simulink model "foc_7"  (R2024a)
settings: Solver=FixedStepAuto  StartTime=0.0  StopTime=3  FixedStep=1e-6  MaxStep=1e-5  RelTol=1e-3
undefined symbols (not defined in the file): DiscIntNeverNeededParam, Ki, Ki_s, Kp, Kp_s, L, lambda, ma, p, R, T_period, Vdc
libraries: simulink x13, spsIGBTDiodeLib x6, spsSeriesRLCBranchLib x6, eeGeneralControl x6, spsCurrentMeasurementLib x3, spsPermanentMagnetSynchronousMachineLib x2, spsDCVoltageSourceLib x1, spsStairGeneratorLib x1, spspowerguiLib x1
(part 2 of 2)

== system foc_7/Subsystem2/Subsystem5/Limitations ==
  Vq_ref1 : Inport
  Vd_ref1 : Inport  Port=2
  Action Port : ActionPort  ActionPortLabel=else
  Add : Sum
  Gain : Gain  Gain=sqrt(3)
  Gain1 : Gain  Gain=Vdc*ma
  Gain2 : Gain  Gain=Vdc*ma
  Product : Product  Inputs=*/
  Product1 : Product  Inputs=/*
  Sqrt : Sqrt
  Square : Math  Operator=square  SignedPower=on
  Square1 : Math  Operator=square  SignedPower=on
  Vq_ref2 : Outport
  Vd_ref2 : Outport  Port=2
  wires:
  Vq_ref1/1 -> Gain2/1, Square/1
  Vd_ref1/1 -> Gain1/1, Square1/1
  Square/1 -> Add/1
  Square1/1 -> Add/2
  Add/1 -> Sqrt/1
  Sqrt/1 -> Gain/1
  Gain2/1 -> Product/1
  Gain1/1 -> Product1/2
  Gain/1 -> Product/2, Product1/1
  Product/1 -> Vq_ref2/1
  Product1/1 -> Vd_ref2/1

== system foc_7/Subsystem2/Subsystem5/Linear Operation  ==
  Vq_ref1 : Inport
  Vd_ref1 : Inport  Port=2
  Action Port : ActionPort  ActionPortLabel=if(u1 <= 0)
  Vq_ref2 : Outport
  Vd_ref2 : Outport  Port=2
  wires:
  Vq_ref1/1 -> Vq_ref2/1
  Vd_ref1/1 -> Vd_ref2/1

== system foc_7/Subsystem3/SVPWM/ABC to alpha-beta ==
  In1 : Inport
  In2 : Inport  Port=2
  In3 : Inport  Port=3
  Add : Sum  Inputs=+--
  Add1 : Sum  Inputs=+-
  Gain : Gain  Gain=0.5
  Gain1 : Gain  Gain=0.5
  Gain2 : Gain  Gain=2/3
  Gain3 : Gain  Gain=sqrt(3)/2
  Gain4 : Gain  Gain=sqrt(3)/2
  Gain5 : Gain  Gain=2/3
  Scope1 : Scope  NumInputPorts=3
  alpha : Outport
  beta : Outport  Port=2
  wires:
  Gain3/1 -> Add1/1
  In2/1 -> Gain3/1, Scope1/2, Gain/1
  Gain4/1 -> Add1/2
  Add1/1 -> Gain5/1
  Gain1/1 -> Add/3
  In3/1 -> Scope1/3, Gain4/1, Gain1/1
  Gain/1 -> Add/2
  In1/1 -> Add/1, Scope1/1
  Add/1 -> Gain2/1
  Gain2/1 -> alpha/1  "alpha"
  Gain5/1 -> beta/1  "beta"

== system foc_7/Subsystem3/SVPWM/PWM ==
  ref1 : Inport
  ref2 : Inport  Port=2
  ref3 : Inport  Port=3
  Carrier : Inport  Port=4
  Relational Operator : RelationalOperator  OutDataTypeStr=boolean  RndMeth=Simplest  InputSameDT=off
  Relational Operator1 : RelationalOperator  OutDataTypeStr=boolean  RndMeth=Simplest  InputSameDT=off
  Relational Operator2 : RelationalOperator  OutDataTypeStr=boolean  RndMeth=Simplest  InputSameDT=off
  PWM1 : Outport
  PWM3 : Outport  Port=2
  PWM5 : Outport  Port=3
  wires:
  ref1/1 -> Relational Operator/1
  ref2/1 -> Relational Operator1/1
  ref3/1 -> Relational Operator2/1
  Carrier/1 -> Relational Operator/2, Relational Operator2/2, Relational Operator1/2
  Relational Operator/1 -> PWM1/1
  Relational Operator1/1 -> PWM3/1
  Relational Operator2/1 -> PWM5/1

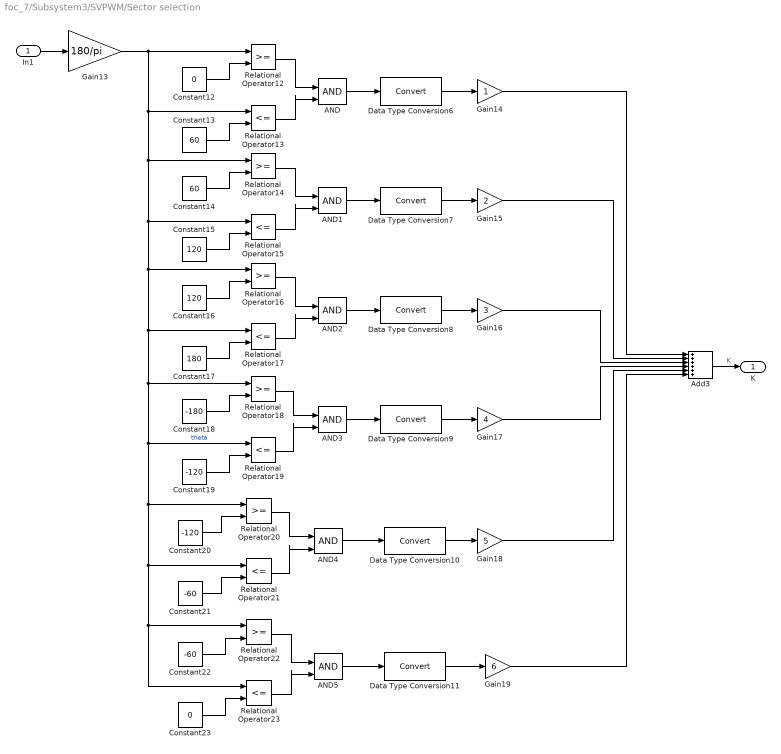
== system foc_7/Subsystem3/SVPWM/Sector selection ==
  In1 : Inport
  AND{,1..5} (6 alike) : Logic  IconShape=distinctive  AllPortsSameDT=off  OutDataTypeStr=boolean
  Add3 : Sum  Inputs=++++++
  Constant12 : Constant  Value=0
  Constant13 : Constant  Value=60
  Constant14 : Constant  Value=60
  Constant15 : Constant  Value=120
  Constant16 : Constant  Value=120
  Constant17 : Constant  Value=180
  Constant18 : Constant  Value=-180
  Constant19 : Constant  Value=-120
  Constant20 : Constant  Value=-120
  Constant21 : Constant  Value=-60
  Constant22 : Constant  Value=-60
  Constant23 : Constant  Value=0
  Data Type Conversion{6..11} (6 alike) : DataTypeConversion  SaturateOnIntegerOverflow=off  RndMeth=Floor
  Gain13 : Gain  Gain=180/pi
  Gain14 : Gain
  Gain15 : Gain  Gain=2
  Gain16 : Gain  Gain=3
  Gain17 : Gain  Gain=4
  Gain18 : Gain  Gain=5
  Gain19 : Gain  Gain=6
  Relational Operator{12,14,16,18,20,22} (6 alike) : RelationalOperator  OutDataTypeStr=boolean  RndMeth=Simplest  InputSameDT=off
  Relational Operator{13,15,17,19,21,23} (6 alike) : RelationalOperator  Operator=<=  OutDataTypeStr=boolean  RndMeth=Simplest  InputSameDT=off
  K : Outport
  wires:
  AND2/1 -> Data Type Conversion8/1
  Relational Operator14/1 -> AND1/1
  Relational Operator12/1 -> AND/1
  Data Type Conversion10/1 -> Gain18/1
  Data Type Conversion8/1 -> Gain16/1
  Relational Operator19/1 -> AND3/2
  Gain13/1 -> Relational Operator14/1, Relational Operator18/1, Relational Operator19/1, Relational Operator20/1, Relational Operator22/1, Relational Operator23/1, Relational Operator21/1, Relational Operator17/1, Relational Operator16/1, Relational Operator15/1, Relational Operator13/1, Relational Operator12/1  "theta"
  Data Type Conversion6/1 -> Gain14/1
  Constant21/1 -> Relational Operator21/2
  Constant19/1 -> Relational Operator19/2
  Gain19/1 -> Add3/6
  Constant18/1 -> Relational Operator18/2
  AND4/1 -> Data Type Conversion10/1
  Constant22/1 -> Relational Operator22/2
  Relational Operator22/1 -> AND5/1
  Relational Operator18/1 -> AND3/1
  Gain15/1 -> Add3/2
  Relational Operator23/1 -> AND5/2
  Data Type Conversion11/1 -> Gain19/1
  Constant16/1 -> Relational Operator16/2
  Data Type Conversion7/1 -> Gain15/1
  Constant23/1 -> Relational Operator23/2
  Relational Operator20/1 -> AND4/1
  Gain18/1 -> Add3/5
  Gain14/1 -> Add3/1
  AND1/1 -> Data Type Conversion7/1
  Constant14/1 -> Relational Operator14/2
  Relational Operator16/1 -> AND2/1
  Relational Operator17/1 -> AND2/2
  Gain17/1 -> Add3/4
  Constant12/1 -> Relational Operator12/2
  Gain16/1 -> Add3/3
  Relational Operator13/1 -> AND/2
  Relational Operator15/1 -> AND1/2
  Data Type Conversion9/1 -> Gain17/1
  AND/1 -> Data Type Conversion6/1
  Constant13/1 -> Relational Operator13/2
  Relational Operator21/1 -> AND4/2
  AND3/1 -> Data Type Conversion9/1
  Constant20/1 -> Relational Operator20/2
  Constant17/1 -> Relational Operator17/2
  AND5/1 -> Data Type Conversion11/1
  Constant15/1 -> Relational Operator15/2
  Add3/1 -> K/1  "K"
  In1/1 -> Gain13/1

== system foc_7/Subsystem3/SVPWM/Subsystem3 ==
  In1 : Inport
  In2 : Inport  Port=2
  In3 : Inport  Port=3
  Add10 : Sum
  Add8 : Sum  Inputs=+++
  Add9 : Sum
  Gain{9..12} (4 alike) : Gain  Gain=0.5
  S1 : Outport
  S3 : Outport  Port=2
  S6 : Outport  Port=3
  S5 : Outport  Port=4
  wires:
  In3/1 -> Gain9/1, Gain10/1, Gain12/1, Gain11/1
  Gain11/1 -> Add10/2
  Gain9/1 -> Add8/3
  Gain10/1 -> Add9/2
  Add8/1 -> S1/1  "S1"
  In2/1 -> Add9/1, Add8/2
  In1/1 -> Add10/1, Add8/1
  Add9/1 -> S3/1  "S3"
  Gain12/1 -> S5/1  "S5"
  Add10/1 -> S6/1  "S6"

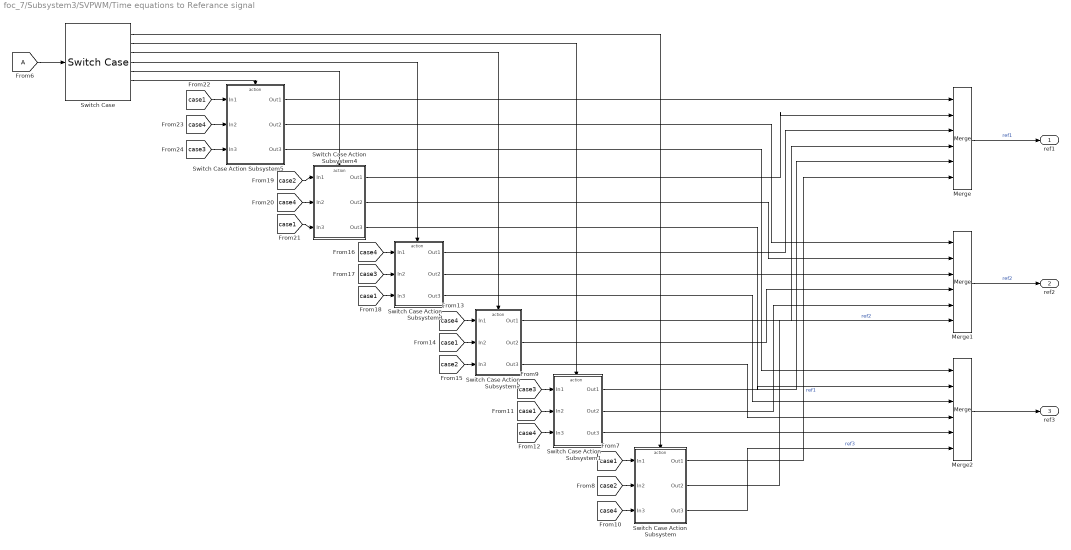
== system foc_7/Subsystem3/SVPWM/Time equations to Referance signal ==
  From6 : From  TagVisibility=global
  Merge : Merge  Inputs=6
  Merge1 : Merge  Inputs=6
  Merge2 : Merge  Inputs=6
  Switch Case : SwitchCase  CaseConditions={1 2 3 4 5 6}
  Switch Case Action Subsystem : Subsystem  TreatAsAtomicUnit=on
  Switch Case Action Subsystem1 : Subsystem  TreatAsAtomicUnit=on
  Switch Case Action Subsystem2 : Subsystem  TreatAsAtomicUnit=on
  Switch Case Action Subsystem3 : Subsystem  TreatAsAtomicUnit=on
  Switch Case Action Subsystem4 : Subsystem  TreatAsAtomicUnit=on
  Switch Case Action Subsystem5 : Subsystem  TreatAsAtomicUnit=on
  ref1 : Outport
  "ref2 " : Outport  Port=2
  ref3 : Outport  Port=3
  wires:
  [case3] -> Switch Case Action Subsystem5/3(In3)
  Switch Case Action Subsystem4/1(Out1) -> Merge/2
  [case1] -> Switch Case Action Subsystem2/2(In2)
  Switch Case Action Subsystem3/2(Out2) -> Merge1/3
  [case4] -> Switch Case Action Subsystem3/1(In1)
  Switch Case/4 -> Switch Case Action Subsystem3/Action
  [case2] -> Switch Case Action Subsystem4/1(In1)
  Switch Case/6 -> Switch Case Action Subsystem5/Action
  [case4] -> Switch Case Action Subsystem1/3(In3)
  [case1] -> Switch Case Action Subsystem5/1(In1)
  [case3] -> Switch Case Action Subsystem1/1(In1)
  Merge/1 -> ref1/1  "ref1"
  Switch Case Action Subsystem5/1(Out1) -> Merge/1
  Switch Case/5 -> Switch Case Action Subsystem4/Action
  Switch Case Action Subsystem4/3(Out3) -> Merge2/2
  [case1] -> Switch Case Action Subsystem/1(In1)
  Switch Case Action Subsystem2/3(Out3) -> Merge2/4
  Switch Case Action Subsystem4/2(Out2) -> Merge1/2
  Switch Case/3 -> Switch Case Action Subsystem2/Action
  Switch Case Action Subsystem/2(Out2) -> Merge1/6  "ref2"
  Switch Case Action Subsystem3/3(Out3) -> Merge2/3
  Switch Case Action Subsystem5/2(Out2) -> Merge1/1
  [case3] -> Switch Case Action Subsystem3/2(In2)
  Switch Case/2 -> Switch Case Action Subsystem1/Action
  Switch Case Action Subsystem2/1(Out1) -> Merge/4
  Switch Case Action Subsystem2/2(Out2) -> Merge1/4
  [case1] -> Switch Case Action Subsystem4/3(In3)
  [case4] -> Switch Case Action Subsystem5/2(In2)
  Switch Case/1 -> Switch Case Action Subsystem/Action
  Switch Case Action Subsystem5/3(Out3) -> Merge2/1
  [case4] -> Switch Case Action Subsystem2/1(In1)
  Switch Case Action Subsystem3/1(Out1) -> Merge/3
  [case4] -> Switch Case Action Subsystem/3(In3)
  Merge2/1 -> ref3/1
  From6/1 -> Switch Case/1
  [case4] -> Switch Case Action Subsystem4/2(In2)
  [case2] -> Switch Case Action Subsystem/2(In2)
  [case2] -> Switch Case Action Subsystem2/3(In3)
  [case1] -> Switch Case Action Subsystem3/3(In3)
  Switch Case Action Subsystem1/2(Out2) -> Merge1/5
  Switch Case Action Subsystem/1(Out1) -> Merge/6  "ref1"
  Switch Case Action Subsystem1/1(Out1) -> Merge/5
  Switch Case Action Subsystem/3(Out3) -> Merge2/6  "ref3"
  Switch Case Action Subsystem1/3(Out3) -> Merge2/5
  [case1] -> Switch Case Action Subsystem1/2(In2)
  Merge1/1 -> "ref2 "/1  "ref2"

== system foc_7/Subsystem3/SVPWM/polar form ==
  In1 : Inport
  In2 : Inport  Port=2
  Add2 : Sum
  Atan2 : Trigonometry  Operator=atan2
  Math Function : Math  Operator=square  SignedPower=on
  Math Function1 : Math  Operator=square  SignedPower=on
  Saturation2 : Saturate  UpperLimit=0.95 * Vdc /sqrt(3)  LowerLimit=0
  Scope1 : Scope  NumInputPorts=2
  Scope2 : Scope  NumInputPorts=2
  Square Root : Sqrt
  Vr : Outport
  Angle : Outport  Port=2
  wires:
  In2/1 -> Scope2/2, Atan2/2, Math Function1/1
  In1/1 -> Scope2/1, Atan2/1, Math Function/1
  Math Function1/1 -> Add2/2
  Add2/1 -> Square Root/1
  Math Function/1 -> Add2/1
  Atan2/1 -> Angle/1
  Square Root/1 -> Saturation2/1, Scope1/1  "Vr"
  Saturation2/1 -> Vr/1, Scope1/2

== system foc_7/Subsystem3/SVPWM/time equations ==
  Vref : Inport
  Sector : Inport  Port=2
  Angle : Inport  Port=3
  Add4 : Sum  Inputs=+-
  Add5 : Sum  Inputs=+-
  Add6 : Sum  Inputs=+-
  Add7 : Sum  Inputs=+--
  Constant : Constant  Value=T_period
  Divide : Product  Inputs=*/
  Gain6 : Gain  Gain=sqrt(3)*(T_period)
  Gain7 : Gain  Gain=pi/3
  Gain8 : Gain  Gain=pi/3
  Product : Product
  Product1 : Product
  Sin1 : Trigonometry
  Sin4 : Trigonometry
  Vdc : Constant  Value=Vdc
  const : Constant
  T1 : Outport
  T2 : Outport  Port=2
  T0 : Outport  Port=3
  wires:
  Vdc/1 -> Divide/2
  Gain6/1 -> Product1/1, Product/1
  Divide/1 -> Gain6/1
  Add6/1 -> Gain8/1
  Constant/1 -> Add7/1
  Gain7/1 -> Add4/1
  Add5/1 -> Sin4/1
  Sin4/1 -> Product1/2
  Sin1/1 -> Product/2
  Gain8/1 -> Add5/2
  Angle/1 -> Add5/1, Add4/2
  const/1 -> Add6/2
  Product1/1 -> T2/1, Add7/3  "T2"
  Sector/1 -> Gain7/1, Add6/1
  Add4/1 -> Sin1/1
  Vref/1 -> Divide/1
  Product/1 -> Add7/2, T1/1  "T1"
  Add7/1 -> T0/1

== system foc_7/Subsystem3/Subsystem2/PI_Controller_Id ==
  Id_error : Inport
  Discrete-Time Integrator1 : DiscreteIntegrator  SampleTime=-1  ICPrevOutput=DiscIntNeverNeededParam  ICPrevScaledInput=DiscIntNeverNeededParam
  Gain1 : Gain  Gain=Kp
  Gain2 : Gain  Gain=Ki
  Product : Product
  Scope : Scope  NumInputPorts=2
  Scope1 : Scope
  Sum1 : Sum
  Vd_coupled : Outport
  wires:
  [Stop_d_integrator] -> Scope/2, Product/1
  Sum1/1 -> Scope1/1, Vd_coupled/1
  Product/1 -> Scope/1, Discrete-Time Integrator1/1
  Gain2/1 -> Product/2
  Discrete-Time Integrator1/1 -> Sum1/2
  Gain1/1 -> Sum1/1
  Id_error/1 -> Gain2/1, Gain1/1

== system foc_7/Subsystem3/Subsystem2/PI_Controller_Iq ==
  Iq_error : Inport
  Discrete-Time Integrator1 : DiscreteIntegrator  SampleTime=-1  ICPrevOutput=DiscIntNeverNeededParam  ICPrevScaledInput=DiscIntNeverNeededParam
  Gain1 : Gain  Gain=Kp
  Gain2 : Gain  Gain=Ki
  Product : Product
  Scope : Scope  NumInputPorts=2
  Scope1 : Scope
  Sum1 : Sum
  Vq_coupled : Outport
  wires:
  Product/1 -> Scope/1, Discrete-Time Integrator1/1
  Iq_error/1 -> Gain2/1, Gain1/1
  Discrete-Time Integrator1/1 -> Sum1/2
  Gain1/1 -> Sum1/1
  Gain2/1 -> Product/2
  [Stop_q_integrator] -> Scope/2, Product/1
  Sum1/1 -> Scope1/1, Vq_coupled/1

== system foc_7/Subsystem3/Subsystem5/Limitations ==
  Vq_ref1 : Inport
  Vd_ref1 : Inport  Port=2
  Action Port : ActionPort
  Add : Sum
  Gain : Gain  Gain=sqrt(3)
  Gain1 : Gain  Gain=Vdc*ma
  Gain2 : Gain  Gain=Vdc*ma
  Product : Product  Inputs=*/
  Product1 : Product  Inputs=/*
  Sqrt : Sqrt
  Square : Math  Operator=square  SignedPower=on
  Square1 : Math  Operator=square  SignedPower=on
  Vq_ref2 : Outport
  Vd_ref2 : Outport  Port=2
  wires:
  Vq_ref1/1 -> Gain2/1, Square/1
  Vd_ref1/1 -> Gain1/1, Square1/1
  Square/1 -> Add/1
  Square1/1 -> Add/2
  Add/1 -> Sqrt/1
  Sqrt/1 -> Gain/1
  Gain2/1 -> Product/1
  Gain1/1 -> Product1/2
  Gain/1 -> Product/2, Product1/1
  Product/1 -> Vq_ref2/1
  Product1/1 -> Vd_ref2/1

== system foc_7/Subsystem3/Subsystem5/Linear Operation  ==
  Vq_ref1 : Inport
  Vd_ref1 : Inport  Port=2
  Action Port : ActionPort
  Vq_ref2 : Outport
  Vd_ref2 : Outport  Port=2
  wires:
  Vq_ref1/1 -> Vq_ref2/1
  Vd_ref1/1 -> Vd_ref2/1

== system foc_7/Subsystem2/SVPWM/Time equations to Referance signal/Switch Case Action Subsystem ==
  In1 : Inport
  In2 : Inport  Port=2
  In3 : Inport  Port=3
  Action Port : ActionPort  ActionPortLabel=case [ 1 ]:
  Out1 : Outport
  Out2 : Outport  Port=2
  Out3 : Outport  Port=3
  wires:
  In1/1 -> Out1/1
  In2/1 -> Out2/1
  In3/1 -> Out3/1

== system foc_7/Subsystem2/SVPWM/Time equations to Referance signal/Switch Case Action Subsystem1 ==
  In1 : Inport
  In2 : Inport  Port=2
  In3 : Inport  Port=3
  Action Port : ActionPort  ActionPortLabel=case [ 2 ]:
  Out1 : Outport
  Out2 : Outport  Port=2
  Out3 : Outport  Port=3
  wires:
  In1/1 -> Out1/1
  In2/1 -> Out2/1
  In3/1 -> Out3/1

== system foc_7/Subsystem2/SVPWM/Time equations to Referance signal/Switch Case Action Subsystem2 ==
  In1 : Inport
  In2 : Inport  Port=2
  In3 : Inport  Port=3
  Action Port : ActionPort  ActionPortLabel=case [ 3 ]:
  Out1 : Outport
  Out2 : Outport  Port=2
  Out3 : Outport  Port=3
  wires:
  In1/1 -> Out1/1
  In2/1 -> Out2/1
  In3/1 -> Out3/1

== system foc_7/Subsystem2/SVPWM/Time equations to Referance signal/Switch Case Action Subsystem3 ==
  In1 : Inport
  In2 : Inport  Port=2
  In3 : Inport  Port=3
  Action Port : ActionPort  ActionPortLabel=case [ 4 ]:
  Out1 : Outport
  Out2 : Outport  Port=2
  Out3 : Outport  Port=3
  wires:
  In1/1 -> Out1/1
  In2/1 -> Out2/1
  In3/1 -> Out3/1

== system foc_7/Subsystem2/SVPWM/Time equations to Referance signal/Switch Case Action Subsystem4 ==
  In1 : Inport
  In2 : Inport  Port=2
  In3 : Inport  Port=3
  Action Port : ActionPort  ActionPortLabel=case [ 5 ]:
  Out1 : Outport
  Out2 : Outport  Port=2
  Out3 : Outport  Port=3
  wires:
  In1/1 -> Out1/1
  In2/1 -> Out2/1
  In3/1 -> Out3/1

== system foc_7/Subsystem2/SVPWM/Time equations to Referance signal/Switch Case Action Subsystem5 ==
  In1 : Inport
  In2 : Inport  Port=2
  In3 : Inport  Port=3
  Action Port : ActionPort  ActionPortLabel=case [ 6 ]:
  Out1 : Outport
  Out2 : Outport  Port=2
  Out3 : Outport  Port=3
  wires:
  In1/1 -> Out1/1
  In2/1 -> Out2/1
  In3/1 -> Out3/1

== system foc_7/Subsystem3/SVPWM/Time equations to Referance signal/Switch Case Action Subsystem ==
  In1 : Inport
  In2 : Inport  Port=2
  In3 : Inport  Port=3
  Action Port : ActionPort
  Out1 : Outport
  Out2 : Outport  Port=2
  Out3 : Outport  Port=3
  wires:
  In1/1 -> Out1/1
  In2/1 -> Out2/1
  In3/1 -> Out3/1

== system foc_7/Subsystem3/SVPWM/Time equations to Referance signal/Switch Case Action Subsystem1 ==
  In1 : Inport
  In2 : Inport  Port=2
  In3 : Inport  Port=3
  Action Port : ActionPort
  Out1 : Outport
  Out2 : Outport  Port=2
  Out3 : Outport  Port=3
  wires:
  In1/1 -> Out1/1
  In2/1 -> Out2/1
  In3/1 -> Out3/1

== system foc_7/Subsystem3/SVPWM/Time equations to Referance signal/Switch Case Action Subsystem2 ==
  In1 : Inport
  In2 : Inport  Port=2
  In3 : Inport  Port=3
  Action Port : ActionPort
  Out1 : Outport
  Out2 : Outport  Port=2
  Out3 : Outport  Port=3
  wires:
  In1/1 -> Out1/1
  In2/1 -> Out2/1
  In3/1 -> Out3/1

== system foc_7/Subsystem3/SVPWM/Time equations to Referance signal/Switch Case Action Subsystem3 ==
  In1 : Inport
  In2 : Inport  Port=2
  In3 : Inport  Port=3
  Action Port : ActionPort
  Out1 : Outport
  Out2 : Outport  Port=2
  Out3 : Outport  Port=3
  wires:
  In1/1 -> Out1/1
  In2/1 -> Out2/1
  In3/1 -> Out3/1

== system foc_7/Subsystem3/SVPWM/Time equations to Referance signal/Switch Case Action Subsystem4 ==
  In1 : Inport
  In2 : Inport  Port=2
  In3 : Inport  Port=3
  Action Port : ActionPort
  Out1 : Outport
  Out2 : Outport  Port=2
  Out3 : Outport  Port=3
  wires:
  In1/1 -> Out1/1
  In2/1 -> Out2/1
  In3/1 -> Out3/1

== system foc_7/Subsystem3/SVPWM/Time equations to Referance signal/Switch Case Action Subsystem5 ==
  In1 : Inport
  In2 : Inport  Port=2
  In3 : Inport  Port=3
  Action Port : ActionPort
  Out1 : Outport
  Out2 : Outport  Port=2
  Out3 : Outport  Port=3
  wires:
  In1/1 -> Out1/1
  In2/1 -> Out2/1
  In3/1 -> Out3/1

== matlab function foc_7/MATLAB Function1 ==
  data: u input; A output; B output
function [A, B] = fcn(u)
% Real quadrature encoder (2000 PPR) simulation with correct direction handling
% A leads B in CW (positive rotation)
% B leads A in CCW (negative rotation)
% Starts with A = B = 0

    persistent u_prev state angle_sum
    if isempty(u_prev)
        u_prev = u;
        state = 0;  % Start at state 0: A=0, B=0
        angle_sum = 0;  % Sum of angles for continuous tracking
        A = 0;
        B = 0;
        return;
    end

    % Encoder parameters
    PPR = 2000;
    step_size = (2*pi) / (PPR * 4);  % 4 states per pulse

    % Update angle sum continuously (supports small movements)
    angle_sum = angle_sum + (u - u_prev);  % Accumulate change in angle
    u_prev = u;

    % Calculate how many full steps we have moved
    steps = floor(angle_sum / step_size);
    
    % Update state with wrap-around (0 to 3)
    state = mod(state + steps, 4);  % 4 quadrature states

    % Reduce the angle sum by the number of full steps to avoid overflow
    angle_sum = angle_sum - steps * step_size;

    % Quadrature lookup table [A, B]
    quad_table = [ ...
        0 0;  % State 0
        1 0;  % State 1
        1 1;  % State 2
        0 1;  % State 3
    ];

    % Output the current A/B signal
    A = quad_table(state + 1, 1);
    B = quad_table(state + 1, 2);
end
